simulink model "Tutorial23"  (R2020a)
settings: Solver=FixedStepDiscrete  StartTime=0.0  StopTime=10.0  FixedStep=1  RelTol=1e-3
libraries: simulink x2
settings Model: Creator=ashok  LastModifiedBy=ashok

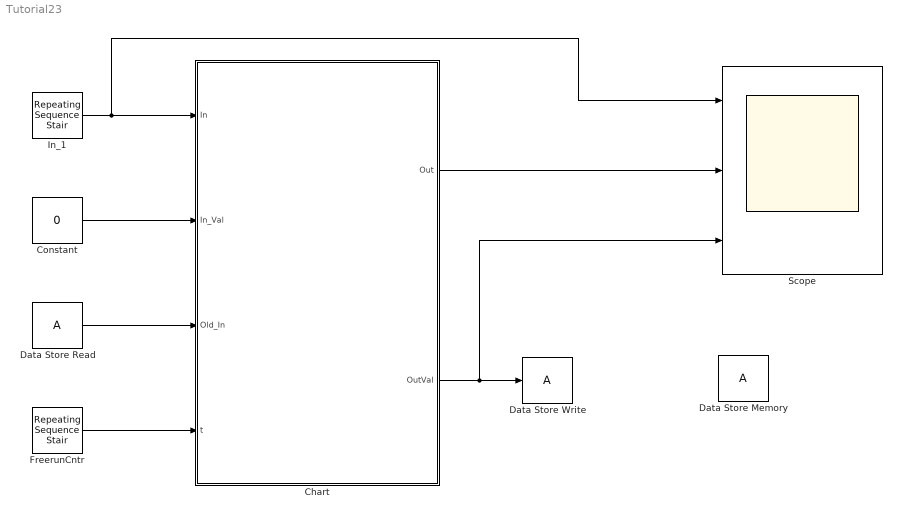
== system Tutorial23 ==
  Chart : Stateflow chart  TreatAsAtomicUnit=on
  Constant : Constant  Value=0
  Data Store Read : DataStoreRead
  Data Store Write : DataStoreWrite
  Data Store Memory : DataStoreMemory  ReadBeforeWriteMsg=warning  WriteAfterWriteMsg=warning  WriteAfterReadMsg=warning  ShowAdditionalParam=off
  FreerunCntr : simulink/Sources/Repeating Sequence Stair  OutValues=FreerunCntr  tsamp=-1  OutMin=[]  OutMax=[]  OutDataTypeStr=double  OutputDataTypeScalingMode=double  OutDataType=fixdt(0,8)  ConRadixGroup=Best Precision: Vector-wise  OutScaling=2^-12
  In_1 : simulink/Sources/Repeating Sequence Stair  OutValues=In_1  tsamp=-1  OutMin=[]  OutMax=[]  OutDataTypeStr=double  OutputDataTypeScalingMode=double  OutDataType=fixdt(0,8)  ConRadixGroup=Best Precision: Vector-wise  OutScaling=2^-12
  Scope : Scope  NumInputPorts=3
  wires:
  In_1/1 -> Scope/1, Chart/1(In)
  Constant/1 -> Chart/2(In_Val)
  Data Store Read/1 -> Chart/3(Old_In)
  FreerunCntr/1 -> Chart/4(t)
  Chart/2(OutVal) -> Scope/3, Data Store Write/1
  Chart/1(Out) -> Scope/2

== stateflow chart Tutorial23/Chart ==
  (default) -> (junction 7)
  (junction 7) -> (junction 10) [order 1] : [t==1]
  (junction 7) -> (junction 9) [order 2] : {
      |    Out = Old_In;
      |    OutVal = In;
      | }
  (junction 10) -> (junction 13) : {
      |   Out = Old_In;
      |   OutVal = In;
      | }
  (junction 13) -> (junction 9)
  (junction 9) -> (junction 16)
  data: In input; In_Val input; Old_In input; t input; Out output; OutVal output
